simulink model "equalizer"  (R2016b)
settings: Solver=VariableStepAuto  StartTime=0.0  StopTime=100  RelTol=1e-3  EnableMultiTasking=on
libraries: dspmathops x3, dspvision x1, dspobslib x1
settings Model: Creator=vladimir_leonidov  LastModifiedBy=vladimir_leonidov
settings DataIOCC: LimitDataPoints=on
settings OptimizationCC: LifeSpan=inf
settings DebuggingCC: AllowSymbolicDim=off  SFUnexpectedBacktrackingDiag=warning  SFNoUnconditionalDefaultTransitionDiag=warning  SFExecutionAtInitializationDiag=none
settings ModelReferenceCC: PropagateSignalLabelsOutOfModel=off
settings GRTTargetCC: TargetLangStandard=C89/C90 (ANSI)
settings ConfigComp: CovMetricSettings=dw  CovHtmlReporting=on  CovSaveCumulativeToWorkspaceVar=on  CovSaveSingleToWorkspaceVar=on  CovExternalEMLEnable=off

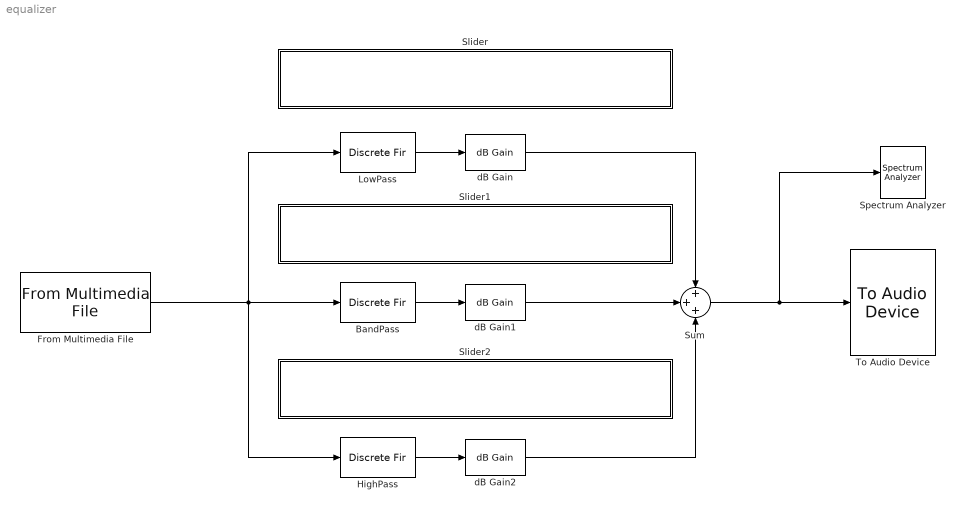
== system equalizer ==
  BandPass : DiscreteFir  Tag=BlockMethodSubSystem  Coefficients=[9.37919605679821675e-05 0.00122577457123756095 0.0023477408870096173 -0.000190033516068428701 -0.00577044623843056981 -0.00566426578724808869 0.00392332904798554753 0.0107525622050162351 0.00360292116357024527 -0.00719919819439160912 -0.00619649841717446245 0.000695425690893493515 0.000126647486629076901 -0.00241150469167185702 0.00277693862756997261 0.00683533370085519319 0.00127553599663492688 -0.00318972223607713037 -9.21433098409217202e-05 -0.000518344043877486723 -0.00606272482686087341 -0.00367370529749674749 0.00417735032309402357 0.00349839211376866627 -0.000265287318958611811 0.00409448691457145637 0.00579794673208390305 -0.00340775984621751338 -0.00761766054555883775 -0.00112546860772881163 -0.000964815489665429675 -0.00623989001470783445 0.000848533409448408394 0.0110924785521314736 0.00540561043183735747 -0.00202787337239356859 0.00354903972825222755 0.00231177225120107093 -0.0121373552140201634 -0.012098835485409451 0.0026920577465470415 0.00267411479479581901 -0.00356890654155190157 0.0097031109828719167 0.0191733033162178566 0.00106434359218114021 -0.0110976917501876705 -0.00025868626047987226 -0.0045894192552380737 -0.0234559974952306856 -0.0100393359340736014 0.0186808163841219871 0.0120549990939827281 0.000167452778267013777 0.0217380834583143986 0.0229664783561496742 -0.0214994455152883179 -0.0342684162052915783 -0.00302029004873356809 -0.0117082073907119767 -0.0366877781558249405 0.0153966907441100836 0.0731980237319985877 0.0284015796019412813 -0.00965513138474943799 0.0471787571289461055 0.0092998084058205175 -0.190379494140850036 -0.207027482835097393 0.121368387039779285 0.348896955804280318 0.121368387039779285 -0.207027482835097393 -0.190379494140850036 0.0092998084058205175 0.0471787571289461055 -0.00965513138474943799 0.0284015796019412813 0.0731980237319985877 0.0153966907441100836 -0.0366877781558249405 -0.0117082073907119767 -0.00302029004873356809 -0.0342684162052915783 -0.0214994455152883179 0.0229664783561496742 0.0217380834583143986 0.000167452778267013777 0.0120549990939827281 0.0186808163841219871 -0.0100393359340736014 -0.0234559974952306856 -0.0045894192552380737 -0.00025868626047987226 -0.0110976917501876705 0.00106434359218114021 0.0191733033162178566 0.0097031109828719167 -0.00356890654155190157 0.00267411479479581901 0.0026920577465470415 -0.012098835485409451 -0.0121373552140201634 0.00231177225120107093 0.00354903972825222755 -0.00202787337239356859 0.00540561043183735747 0.0110924785521314736 0.000848533409448408394 -0.00623989001470783445 -0.000964815489665429675 -0.00112546860772881163 -0.00761766054555883775 -0.00340775984621751338 0.00579794673208390305 0.00409448691457145637 -0.000265287318958611811 0.00349839211376866627 0.00417735032309402357 -0.00367370529749674749 -0.00606272482686087341 -0.000518344043877486723 -9.21433098409217202e-05 -0.00318972223607713037 0.00127553599663492688 0.00683533370085519319 0.00277693862756997261 -0.00241150469167185702 0.000126647486629076901 0.000695425690893493515 -0.00619649841717446245 -0.00719919819439160912 0.00360292116357024527 0.0107525622050162351 0.00392332904798554753 -0.00566426578724808869 -0.00577044623843056981 -0.000190033516068428701 0.0023477408870096173 0.00122577457123756095 9.37919605679821675e-05]  InputProcessing=Columns as channels (frame based)
  From Multimedia File : dspvision/From Multimedia File  inputFilename=/Users/vladimir_leonidov/Library/Mobile Documents/com~apple~CloudDocs/Matlab Projects/Filters/rock.wav  loop=on  numPlays=inf  outputStreams=Audio only  videoDataType=single  audioDataType=double  inheritSampleTime=on  userDefinedSampleTime=1/30  noAudioOutput=off  isIntensityVideo=off  fourcc=RGB  colorVideoFormat=Separate color signals  outputEOF=off  dataOrg=Column-major  audioFrameSize=1024  computeAudioFrameSize=off  outSamplingMode=Sample based
  HighPass : DiscreteFir  Tag=BlockMethodSubSystem  Coefficients=[0.000363016216841819533 -0.00195981077731224645 0.00484813578231365651 -0.00744837263883381222 0.0070667414575812269 -0.00288653869427886933 -0.0021992300521405969 0.00382032545055593139 -0.000965474604549394289 -0.00250267948620643259 0.00230699742032925608 0.00092486009195951401 -0.0025947338180712788 0.000453352272456172009 0.00227212193478957278 -0.00154150469184927597 -0.00154606233090527818 0.00229816431618093961 0.000520907690925092237 -0.00263911501172580743 0.00067515986484523768 0.00248631188235158649 -0.00186945266999878059 -0.00180437841826570867 0.0028493778427441949 0.000632483045246969673 -0.00338183417256180925 0.000879201027638989432 0.00327120763115128612 -0.00247001656671672933 -0.00242553456039949419 0.00381585159600153923 0.000889268929126583855 -0.00458291616044308354 0.00114111648509814673 0.00449008284675639011 -0.00331870239883496699 -0.00338892601721192113 0.00519373149035685239 0.00132828035566175595 -0.00630425339909573054 0.00143224433829591759 0.00626710056641319874 -0.0044445406570196317 -0.00485914915386170387 0.00711902707076476297 0.0020953776816954729 -0.00881312286435796503 0.00172007251259484982 0.0089596500048608578 -0.00600580785106530606 -0.00719356818028381913 0.00997217680825209125 0.00344936317558675824 -0.0127256998726520496 0.00197515071342328503 0.0134018083817323639 -0.00839775394815679872 -0.0113169662614508084 0.0147922008545421368 0.00610714838703198867 -0.0198820777561773722 0.00217895867377531369 0.0222563266518766567 -0.0130476654599428667 -0.0204562903142970418 0.0255935586969391372 0.0129432302304176659 -0.0385975941314544435 0.00230417099337622278 0.0506781327879375562 -0.0295225724295834005 -0.0604779505906793829 0.0842050385952354957 0.0668602290370743091 -0.310765190551585246 0.43092527536211106 -0.310765190551585246 0.0668602290370743091 0.0842050385952354957 -0.0604779505906793829 -0.0295225724295834005 0.0506781327879375562 0.00230417099337622278 -0.0385975941314544435 0.0129432302304176659 0.0255935586969391372 -0.0204562903142970418 -0.0130476654599428667 0.0222563266518766567 0.00217895867377531369 -0.0198820777561773722 0.00610714838703198867 0.0147922008545421368 -0.0113169662614508084 -0.00839775394815679872 0.0134018083817323639 0.00197515071342328503 -0.0127256998726520496 0.00344936317558675824 0.00997217680825209125 -0.00719356818028381913 -0.00600580785106530606 0.0089596500048608578 0.00172007251259484982 -0.00881312286435796503 0.0020953776816954729 0.00711902707076476297 -0.00485914915386170387 -0.0044445406570196317 0.00626710056641319874 0.00143224433829591759 -0.00630425339909573054 0.00132828035566175595 0.00519373149035685239 -0.00338892601721192113 -0.00331870239883496699 0.00449008284675639011 0.00114111648509814673 -0.00458291616044308354 0.000889268929126583855 0.00381585159600153923 -0.00242553456039949419 -0.00247001656671672933 0.00327120763115128612 0.000879201027638989432 -0.00338183417256180925 0.000632483045246969673 0.0028493778427441949 -0.00180437841826570867 -0.00186945266999878059 0.00248631188235158649 0.00067515986484523768 -0.00263911501172580743 0.000520907690925092237 0.00229816431618093961 -0.00154606233090527818 -0.00154150469184927597 0.00227212193478957278 0.000453352272456172009 -0.0025947338180712788 0.00092486009195951401 0.00230699742032925608 -0.00250267948620643259 -0.000965474604549394289 0.00382032545055593139 -0.0021992300521405969 -0.00288653869427886933 0.0070667414575812269 -0.00744837263883381222 0.00484813578231365651 -0.00195981077731224645 0.000363016216841819533]  InputProcessing=Columns as channels (frame based)
  LowPass : DiscreteFir  Tag=BlockMethodSubSystem  Coefficients=[-1.63357231008043167e-05 -0.000274947116561084456 -0.000689930331549650747 -0.00140422332356177743 -0.00239963287317427687 -0.00359041072849649277 -0.0047918917501154467 -0.00574345388340303728 -0.0061636096514144454 -0.00582981492778883621 -0.00466165498665458648 -0.00277934452327974939 -0.000511367156864577844 0.00166270237391899175 0.00322850607910409428 0.00378462896482213967 0.00317799134330252293 0.00157938533547938948 -0.000535292431408226021 -0.00250523458659571542 -0.00367933407417928189 -0.00362877189289603037 -0.00230702467040223543 -9.64231226226672775e-05 0.00228753218127566906 0.00401573869073800545 0.00442540206519239591 0.00326759426936718087 0.000831766441568441918 -0.00210974662237205972 -0.00453487066162813063 -0.00551680855606797096 -0.0045677144248247167 -0.0018567431520785365 0.00178899591066498552 0.00512239125313097322 0.00689022669424689885 0.00629045447317887717 0.00331013035337476575 -0.00119097462540831804 -0.00570713685808253018 -0.00857262750740070412 -0.0085562322506875562 -0.00535851480937758057 0.000179523827350431446 0.00626219409432448703 0.0106936980382196772 0.0116392436632707461 0.00833864205509289927 0.00150945428486394398 -0.0067405871418781205 -0.0135156710039904208 -0.0160905152080164406 -0.012925614689908051 -0.00438422512075175783 0.00713736321499772435 0.0177832859109571632 0.02340408616035973 0.0209884989349990343 0.00991225673453808263 -0.00743413075684349646 -0.0259148408875643707 -0.0388313085227919436 -0.0397423063019343853 -0.0244238179065030016 0.00761323419075139556 0.0525353193266228924 0.102768954469871332 0.148658647445467196 0.180785592844278753 0.192324225688012468 0.180785592844278753 0.148658647445467196 0.102768954469871332 0.0525353193266228924 0.00761323419075139556 -0.0244238179065030016 -0.0397423063019343853 -0.0388313085227919436 -0.0259148408875643707 -0.00743413075684349646 0.00991225673453808263 0.0209884989349990343 0.02340408616035973 0.0177832859109571632 0.00713736321499772435 -0.00438422512075175783 -0.012925614689908051 -0.0160905152080164406 -0.0135156710039904208 -0.0067405871418781205 0.00150945428486394398 0.00833864205509289927 0.0116392436632707461 0.0106936980382196772 0.00626219409432448703 0.000179523827350431446 -0.00535851480937758057 -0.0085562322506875562 -0.00857262750740070412 -0.00570713685808253018 -0.00119097462540831804 0.00331013035337476575 0.00629045447317887717 0.00689022669424689885 0.00512239125313097322 0.00178899591066498552 -0.0018567431520785365 -0.0045677144248247167 -0.00551680855606797096 -0.00453487066162813063 -0.00210974662237205972 0.000831766441568441918 0.00326759426936718087 0.00442540206519239591 0.00401573869073800545 0.00228753218127566906 -9.64231226226672775e-05 -0.00230702467040223543 -0.00362877189289603037 -0.00367933407417928189 -0.00250523458659571542 -0.000535292431408226021 0.00157938533547938948 0.00317799134330252293 0.00378462896482213967 0.00322850607910409428 0.00166270237391899175 -0.000511367156864577844 -0.00277934452327974939 -0.00466165498665458648 -0.00582981492778883621 -0.0061636096514144454 -0.00574345388340303728 -0.0047918917501154467 -0.00359041072849649277 -0.00239963287317427687 -0.00140422332356177743 -0.000689930331549650747 -0.000274947116561084456 -1.63357231008043167e-05]  InputProcessing=Columns as channels (frame based)
  Slider : Subsystem  DialogController=hmiCreateDDGDialog  IsWebBlock=on  mask(MWDashboardBlock){webBlockId=dd40eb2c-ae44-4d90-9898-2e9f792127c0, webBlockType=slider, ShowInLibBrowser=on, ShowInitialText=on, HMISrcModelName=equalizer}
      mask prompts: webBlockId "WebBlock Id"; webBlockType "WebBlock Type"; HMISrcModelName "Source Model"
      mask help: SimulinkHMI:dialogs:SliderDialogDesc
      mask Help: helpview([docroot '/mapfiles/simulink.map'], 'hmi_slider')
      mask Display:
      | if strcmp(get_param(bdroot(gcb),'BlockDiagramType'), 'library')
      |     image([(matlabroot) '/toolbox/simulink/hmi/icons/Slider.png']);
      | end
  Slider1 : Subsystem  DialogController=hmiCreateDDGDialog  IsWebBlock=on  mask(MWDashboardBlock){webBlockId=b3728e76-50be-4e79-975c-56aa297b48ec, webBlockType=slider, ShowInLibBrowser=on, ShowInitialText=on, HMISrcModelName=equalizer}
      mask prompts: webBlockId "WebBlock Id"; webBlockType "WebBlock Type"; HMISrcModelName "Source Model"
      mask help: SimulinkHMI:dialogs:SliderDialogDesc
      mask Help: helpview([docroot '/mapfiles/simulink.map'], 'hmi_slider')
      mask Display:
      | if strcmp(get_param(bdroot(gcb),'BlockDiagramType'), 'library')
      |     image([(matlabroot) '/toolbox/simulink/hmi/icons/Slider.png']);
      | end
  Slider2 : Subsystem  DialogController=hmiCreateDDGDialog  IsWebBlock=on  mask(MWDashboardBlock){webBlockId=92489b70-a786-4ba8-8b0d-b65989cbc150, webBlockType=slider, ShowInLibBrowser=on, ShowInitialText=on, HMISrcModelName=equalizer}
      mask prompts: webBlockId "WebBlock Id"; webBlockType "WebBlock Type"; HMISrcModelName "Source Model"
      mask help: SimulinkHMI:dialogs:SliderDialogDesc
      mask Help: helpview([docroot '/mapfiles/simulink.map'], 'hmi_slider')
      mask Display:
      | if strcmp(get_param(bdroot(gcb),'BlockDiagramType'), 'library')
      |     image([(matlabroot) '/toolbox/simulink/hmi/icons/Slider.png']);
      | end
  Spectrum Analyzer : SpectrumAnalyzer
  Sum : Sum  Inputs=+++
  To Audio Device : dspobslib/To Audio Device  deviceName=Built-in Output  inheritSampleRate=on  sampleRate=44100  deviceDatatype=Determine from input data type  autoBufferSize=on  bufferSize=4096  queueDuration=1.0  defaultOutputChannelMapping=on  outputChannelMapping=1:2  outputNumUnderrunSamples=off
  dB Gain : dspmathops/dB Gain  dB=0  intype=Amplitude
  dB Gain1 : dspmathops/dB Gain  dB=0  intype=Amplitude
  dB Gain2 : dspmathops/dB Gain  dB=0  intype=Amplitude
  wires:
  dB Gain/1 -> Sum/1
  dB Gain1/1 -> Sum/2
  dB Gain2/1 -> Sum/3
  Sum/1 -> Spectrum Analyzer/1, To Audio Device/1
  HighPass/1 -> dB Gain2/1
  BandPass/1 -> dB Gain1/1
  LowPass/1 -> dB Gain/1
  From Multimedia File/1 -> LowPass/1, HighPass/1, BandPass/1

== system equalizer/Slider ==

== system equalizer/Slider1 ==

== system equalizer/Slider2 ==
